simulink model "ae461starter_lab8"  (R2021a)
settings: Solver=ode1  StartTime=0.0  StopTime=inf  FixedStep=0.001  RelTol=1e-3  EnableMultiTasking=on
values from neighbouring files (symbols this model uses):
  Kd = 6    [analysis.m]    (also in params.m)
  KI = 6    [analysis.m]    (also in params.m)
  Kp = 0.6    [analysis.m]    (also in params.m)
libraries: coecsllib x1
Description:
  | Real-Time Van der Pol Simulation
  | 
  | This demonstration shows a real-time version of the Simulink(R) Van der Pol
  | simulation demo. This model does not need any external signals, so it does
  | not need any data acquisition hardware or driver. This makes the model ideal
  | for first experiments with Real-Time Windows Target(TM), without need to
  | worry about proper I/O hardware configuration.
  | 
  | How to run this demo:
  | 
  |   1. Build the model using Tools -> Real-Time Workshop -> Build Model.
  |   2. Connect to the real-time code using Simulation -> Connect to target.
  |   3. Start the real-time execution using Simulation -> Start real-time code.
settings Model: SimulationMode=external  ExtModeTrigDuration=120000  Creator=Houska  LastModifiedBy=abomrar2
settings SolverCC: AlgebraicLoopSolver=TrustRegion
settings DataIOCC: SaveFormat=Array  SignalLoggingSaveFormat=ModelDataLogs  ReturnWorkspaceOutputs=off  SignalLoggingName=logsOut
settings OptimizationCC: ExpressionDepthLimit=2147483647  InitFltsAndDblsToZero=on  EfficientMapNaN2IntZero=off
settings DebuggingCC: UnderspecifiedInitializationDetection=Classic  MergeDetectMultiDrivingBlocksExec=none  SignalResolutionControl=TryResolveAllWithWarning  FcnCallInpInsideContextMsg=warning  StateNameClashWarn=warning  SFUnexpectedBacktrackingDiag=warning  SFNoUnconditionalDefaultTransitionDiag=warning  SFExecutionAtInitializationDiag=none  SFMachineParentedDataDiag=warning  ArithmeticOperatorsInVariantConditions=warning
settings ModelReferenceCC: PropagateSignalLabelsOutOfModel=off
settings SFSimCC: SimUseLocalCustomCode=off  CustomCodeUndefinedFunction=UseInterfaceOnly
settings RTWCC: Description=Simulink Desktop Real-Time  SystemTargetFile=sldrt.tlc  TemplateMakefile=sldrt.tmf  RTWUseLocalCustomCode=off  RTWCompilerOptimization=on
settings CodeAppCC: MaxIdLength=95  StateflowObjectComments=on
settings SimulinkDesktopRealTimeCC: TargetPreCompLibLocation=C:\MATLABR2021a\toolbox\sldrt\lib\win64  TargetLangStandard=C89/C90 (ANSI)  SupportVariableSizeSignals=off
settings ConfigComp: CovMetricSettings=dw  CovSaveCumulativeToWorkspaceVar=on  CovSaveSingleToWorkspaceVar=on  CovExternalEMLEnable=off  CovSFcnEnable=off

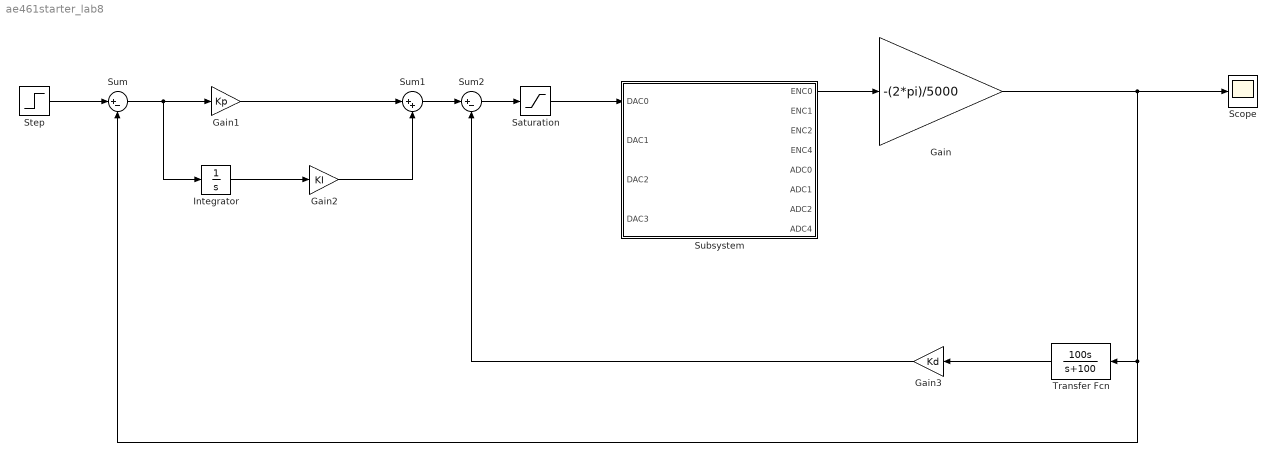
== system ae461starter_lab8 ==
  Gain : Gain  Gain=-(2*pi)/5000
  Gain1 : Gain  Gain=Kp
  Gain2 : Gain  Gain=KI
  Gain3 : Gain  Gain=Kd
  Integrator : Integrator
  Saturation : Saturate  UpperLimit=10  LowerLimit=-10
  Scope : Scope
  Step : Step  Time=0  After=.5  SampleTime=0
  Subsystem : Subsystem
  Sum : Sum  Inputs=|+-
  Sum1 : Sum  Inputs=|++
  Sum2 : Sum  Inputs=|+-
  Transfer Fcn : TransferFcn  Numerator=[100 0]  Denominator=[1 100]
  wires:
  Subsystem/1(ENC0) -> Gain/1
  Saturation/1 -> Subsystem/1(DAC0)
  Step/1 -> Sum/1
  Sum/1 -> Integrator/1, Gain1/1
  Integrator/1 -> Gain2/1
  Gain1/1 -> Sum1/1
  Gain2/1 -> Sum1/2
  Sum1/1 -> Sum2/1
  Sum2/1 -> Saturation/1
  Transfer Fcn/1 -> Gain3/1
  Gain3/1 -> Sum2/2
  Gain/1 -> Scope/1, Sum/2, Transfer Fcn/1

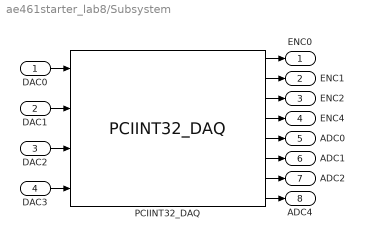
== system ae461starter_lab8/Subsystem ==
  DAC0 : Inport
  DAC1 : Inport  Port=2
  DAC2 : Inport  Port=3
  DAC3 : Inport  Port=4
  PCIINT32_DAQ : coecsllib/Control Systems Lab Board Series/PCIINT32_DAQ  baddr2=findPCIint32BoardAddress3  sampleTime=str2num(get_param(bdroot, 'FixedStep'))
  ENC0 : Outport
  ENC1 : Outport  Port=2
  ENC2 : Outport  Port=3
  ENC4 : Outport  Port=4
  ADC0 : Outport  Port=5
  ADC1 : Outport  Port=6
  ADC2 : Outport  Port=7
  ADC4 : Outport  Port=8
  wires:
  DAC1/1 -> PCIINT32_DAQ/2
  DAC2/1 -> PCIINT32_DAQ/3
  DAC3/1 -> PCIINT32_DAQ/4
  PCIINT32_DAQ/4 -> ENC4/1
  PCIINT32_DAQ/8 -> ADC4/1
  PCIINT32_DAQ/2 -> ENC1/1
  DAC0/1 -> PCIINT32_DAQ/1
  PCIINT32_DAQ/3 -> ENC2/1
  PCIINT32_DAQ/1 -> ENC0/1
  PCIINT32_DAQ/6 -> ADC1/1
  PCIINT32_DAQ/7 -> ADC2/1
  PCIINT32_DAQ/5 -> ADC0/1
